simulink model "mcb_microchip_pmsm_parameter_est_SAME70"  (R2023b)
settings: Solver=FixedStepDiscrete  StartTime=0.0  StopTime=15  RelTol=1e-3  EnableMultiTasking=on
InitFcn:
  | mcb_microchip_pmsm_parameter_est_SAME70_data;
values from neighbouring files (symbols this model uses):
  Ts = T_pwm    (= 5e-05)    [mcb_microchip_pmsm_parameter_est_SAME70_data.m]
  Ts_motor = T_pwm/2    (= 2.5e-05)    [mcb_microchip_pmsm_parameter_est_SAME70_data.m]
undefined symbols (not defined in the file or in its folder): A24, AD10, AD7, ADC0, inverter, LQFP144, MaxPer, ms, ns, PA0, PA1, PA10, PA11, PA12, PA13, PA16, PA18, PA9, PB0, PD18, PD19, PD24, PD25, PD26, PI_params, Pin, pmsm, Resol, SAME70Q21B, target, Unsigned
libraries: simulink x18, MCHP_Blockset x13, mcbpmsmparamestlib x5, svdutilitieslib x4, mcbpositiondecoderlib x3, mcbplantlib x1, autolibpmsmexterior x1, mcbcontrolslib x1
(part 4 of 4)

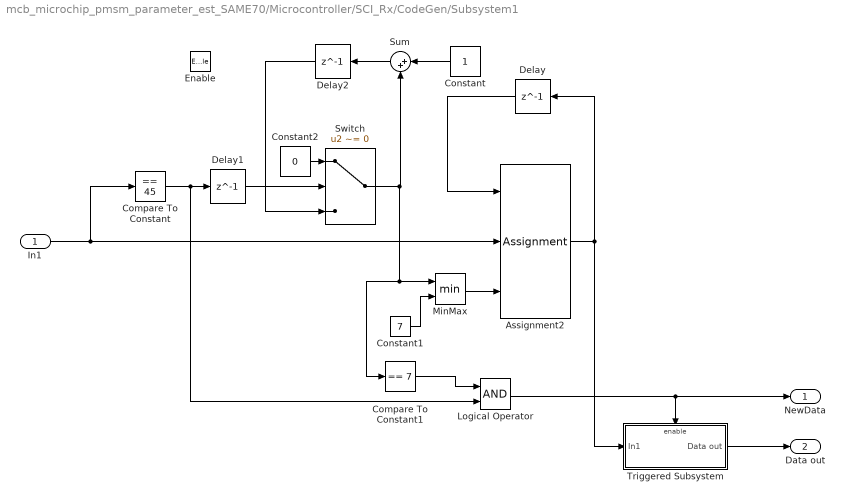
== system mcb_microchip_pmsm_parameter_est_SAME70/Microcontroller/SCI_Rx/CodeGen/Subsystem1 ==
  In1 : Inport
  Enable : EnablePort
  Assignment2 : Assignment  IndexMode=Zero-based  DiagnosticForDimensions=Warning  IndexOptions=Starting index (port)  Indices=1  OutputSizes=1
  Compare To Constant : simulink/Logic and Bit Operations/Compare To Constant  relop===  const=45  OutDataTypeStr=boolean
  Compare To Constant1 : simulink/Logic and Bit Operations/Compare To Constant  relop===  const=7  OutDataTypeStr=boolean
  Constant : Constant  OutDataTypeStr=uint16  SampleTime=-1
  Constant1 : Constant  Value=7  OutDataTypeStr=uint16  SampleTime=-1
  Constant2 : Constant  Value=0  OutDataTypeStr=uint16  SampleTime=-1
  Delay : Delay  DelayLength=1  InitialCondition=[0 0 0 0 0 0 0 0]
  Delay1 : Delay  DelayLength=1  InitialCondition=0
  Delay2 : Delay  DelayLength=1  InitialCondition=0
  Logical Operator : Logic  AllPortsSameDT=off  OutDataTypeStr=boolean
  MinMax : MinMax  Inputs=2
  Sum : Sum  Inputs=|++
  Switch : Switch  Criteria=u2 ~= 0  SaturateOnIntegerOverflow=off  InputSameDT=off
  Triggered Subsystem : Subsystem  TreatAsAtomicUnit=on
  NewData : Outport  OutputWhenDisabled=reset  InitialOutput=0
  Data out : Outport  Port=2
  wires:
  Logical Operator/1 -> Triggered Subsystem/Enable, NewData/1
  Constant2/1 -> Switch/1
  Delay1/1 -> Switch/2
  Switch/1 -> MinMax/1, Compare To Constant1/1, Sum/2
  Sum/1 -> Delay2/1
  MinMax/1 -> Assignment2/3
  Constant1/1 -> MinMax/2
  Constant/1 -> Sum/1
  In1/1 -> Assignment2/2, Compare To Constant/1
  Compare To Constant1/1 -> Logical Operator/1
  Compare To Constant/1 -> Delay1/1, Logical Operator/2
  Delay2/1 -> Switch/3
  Delay/1 -> Assignment2/1
  Assignment2/1 -> Delay/1, Triggered Subsystem/1(In1)
  Triggered Subsystem/1(Data out) -> Data out/1

== system mcb_microchip_pmsm_parameter_est_SAME70/Microcontroller/SCI_Tx/Codegen/Data ==
  Data : Inport
  Action Port : ActionPort  ActionPortLabel=else
  UART Tx : MCHP_Blockset/BUS UART/UART Tx  UART_REF=UART 0  ORDERING=None  AllOrNothing=off  SampleTime=-1  MCHP_MASTERLINK=mcb_microchip_pmsm_parameter_est_SAME70_23b_lib/Microcontroller/Configurations/Microchip Master  NSend_Input=off  UART_String=off  NSend_Output=off
      settings: SourceProductName=MPLAB Device Blocks for Simulink
  wires:
  Data/1 -> UART Tx/1

== system mcb_microchip_pmsm_parameter_est_SAME70/Microcontroller/SCI_Tx/Codegen/End ==
  Data : Inport
  Action Port : ActionPort  ActionPortLabel=elseif(u1 == single(target.SerialFrameSize-1))
  Mux : Mux  Inputs=2
  Start : Constant  Value=hex2dec('45')  OutDataTypeStr=uint8
  UART Tx : MCHP_Blockset/BUS UART/UART Tx  UART_REF=UART 0  ORDERING=None  AllOrNothing=off  SampleTime=-1  MCHP_MASTERLINK=mcb_microchip_pmsm_parameter_est_SAME70_23b_lib/Microcontroller/Configurations/Microchip Master  NSend_Input=off  UART_String=off  NSend_Output=off
      settings: SourceProductName=MPLAB Device Blocks for Simulink
  wires:
  Start/1 -> Mux/2
  Data/1 -> Mux/1
  Mux/1 -> UART Tx/1

== system mcb_microchip_pmsm_parameter_est_SAME70/Microcontroller/SCI_Tx/Codegen/Start ==
  Data : Inport
  Action Port : ActionPort  ActionPortLabel=if(u1 == 0)
  End : Constant  Value=hex2dec('53')  OutDataTypeStr=uint8
  Mux : Mux  Inputs=2
  UART Tx : MCHP_Blockset/BUS UART/UART Tx  UART_REF=UART 0  ORDERING=None  AllOrNothing=off  SampleTime=-1  MCHP_MASTERLINK=mcb_microchip_pmsm_parameter_est_SAME70_23b_lib/Microcontroller/Configurations/Microchip Master  NSend_Input=off  UART_String=off  NSend_Output=off
      settings: SourceProductName=MPLAB Device Blocks for Simulink
  wires:
  End/1 -> Mux/1
  Data/1 -> Mux/2
  Mux/1 -> UART Tx/1

== system mcb_microchip_pmsm_parameter_est_SAME70/Inverter and Motor/Inverter and Motor/Sim/Motor/Inverter ==
  Duty_abc : Inport
  Average-Value Inverter : mcbplantlib/Average-Value Inverter
  Constant2 : Constant  Value=inverter.V_dc  OutDataTypeStr=single  SampleTime=-1
  Data Type Conversion1 : DataTypeConversion  OutDataTypeStr=single  RndMeth=Simplest  SaturateOnIntegerOverflow=off
  Vabc : Outport
  wires:
  Constant2/1 -> Average-Value Inverter/2
  Duty_abc/1 -> Data Type Conversion1/1
  Average-Value Inverter/1 -> Vabc/1
  Data Type Conversion1/1 -> Average-Value Inverter/1

== system mcb_microchip_pmsm_parameter_est_SAME70/Microcontroller/Application/Param Est/MechParam/Select J ==
  Jin : Inport
  codegen : Subsystem  VariantControl=(codegen)
  sim : Subsystem  VariantControl=(sim)
  Jout : Outport

== system mcb_microchip_pmsm_parameter_est_SAME70/Microcontroller/Application Abstraction/Variant Subsystem/Index Absent/Enabled Subsystem ==
  In1 : Inport
  Enable : EnablePort
  Out1 : Outport
  wires:
  In1/1 -> Out1/1

== system mcb_microchip_pmsm_parameter_est_SAME70/Microcontroller/Input HW Drivers/Codegen/Qdec_interface/If Action Subsystem ==
  In1 : Inport
  Action Port : ActionPort  ActionPortLabel=if((u1 > 49151 ) & (u2 < 16384 ))
  Add : Sum
  Constant : Constant  Value=(EnCountPerRev) -mod(65536,(EnCountPerRev))  OutDataTypeStr=uint16
  Out1 : Outport
  wires:
  In1/1 -> Add/1
  Constant/1 -> Add/2
  Add/1 -> Out1/1

== system mcb_microchip_pmsm_parameter_est_SAME70/Microcontroller/Input HW Drivers/Codegen/Qdec_interface/If Action Subsystem1 ==
  In1 : Inport
  Action Port : ActionPort  ActionPortLabel=elseif((u2 > 49151 ) & (u1 < 16384 ))
  Add : Sum
  Constant : Constant  Value=mod(65536,(EnCountPerRev))  OutDataTypeStr=uint16
  Out1 : Outport
  wires:
  Add/1 -> Out1/1
  Constant/1 -> Add/2
  In1/1 -> Add/1

== system mcb_microchip_pmsm_parameter_est_SAME70/Microcontroller/Input HW Drivers/Codegen/Qdec_interface/If Action Subsystem2 ==
  In1 : Inport
  Action Port : ActionPort  ActionPortLabel=else
  Out1 : Outport
  wires:
  In1/1 -> Out1/1

== system mcb_microchip_pmsm_parameter_est_SAME70/Microcontroller/Input HW Drivers/Codegen/Qdec_interface/Offset ==
  QdecCount : Inport
  Enable : EnablePort
  Add1 : Sum  Inputs=-+  OutDataTypeStr=uint16
  Constant2 : Constant  Value=EnCountPerRev  OutDataTypeStr=Inherit: Inherit via back propagation
  Data Store Write : DataStoreWrite  DataStoreName=PosOffset  IndexOptions=Index vector (dialog)  Indices=1  OutputSizes=1
  Math Function1 : Math  Operator=mod  SignedPower=on
  wires:
  QdecCount/1 -> Math Function1/1
  Constant2/1 -> Add1/2, Math Function1/2
  Add1/1 -> Data Store Write/1
  Math Function1/1 -> Add1/1

== system mcb_microchip_pmsm_parameter_est_SAME70/Microcontroller/Input Scaling/Variant Subsystem/Automatic offset calibration/Enabled Subsystem ==
  In1 : Inport
  Enable : EnablePort
  Out1 : Outport
  wires:
  In1/1 -> Out1/1

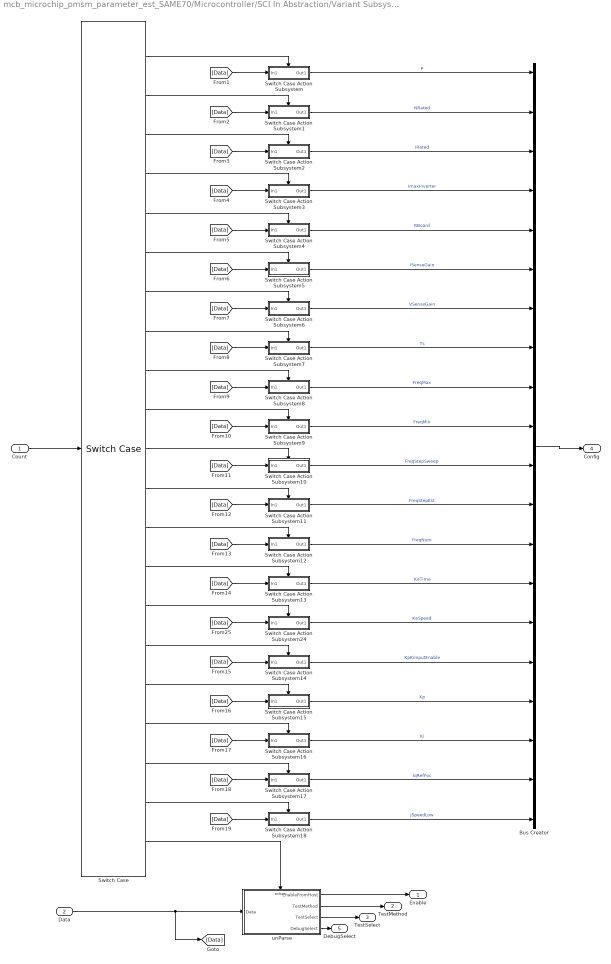
== system mcb_microchip_pmsm_parameter_est_SAME70/Microcontroller/SCI In Abstraction/Variant Subsystem/Codegen/Subsystem1 ==
  Count : Inport
  Data : Inport  Port=2
  Bus Creator : BusCreator  Inputs=20
  Switch Case : SwitchCase  CaseConditions={1 2 3 4 5 6 7 8 9 10 11 12 13 14 15 16 17 18 19 20 21}  ShowDefaultCase=off
  Switch Case Action Subsystem : Subsystem  TreatAsAtomicUnit=on
  Switch Case Action Subsystem1 : Subsystem  TreatAsAtomicUnit=on
  Switch Case Action Subsystem10 : Subsystem  TreatAsAtomicUnit=on
  Switch Case Action Subsystem11 : Subsystem  TreatAsAtomicUnit=on
  Switch Case Action Subsystem12 : Subsystem  TreatAsAtomicUnit=on
  Switch Case Action Subsystem13 : Subsystem  TreatAsAtomicUnit=on
  Switch Case Action Subsystem14 : Subsystem  TreatAsAtomicUnit=on
  Switch Case Action Subsystem15 : Subsystem  TreatAsAtomicUnit=on
  Switch Case Action Subsystem16 : Subsystem  TreatAsAtomicUnit=on
  Switch Case Action Subsystem17 : Subsystem  TreatAsAtomicUnit=on
  Switch Case Action Subsystem18 : Subsystem  TreatAsAtomicUnit=on
  Switch Case Action Subsystem2 : Subsystem  TreatAsAtomicUnit=on
  Switch Case Action Subsystem24 : Subsystem  TreatAsAtomicUnit=on
  Switch Case Action Subsystem3 : Subsystem  TreatAsAtomicUnit=on
  Switch Case Action Subsystem4 : Subsystem  TreatAsAtomicUnit=on
  Switch Case Action Subsystem5 : Subsystem  TreatAsAtomicUnit=on
  Switch Case Action Subsystem6 : Subsystem  TreatAsAtomicUnit=on
  Switch Case Action Subsystem7 : Subsystem  TreatAsAtomicUnit=on
  Switch Case Action Subsystem8 : Subsystem  TreatAsAtomicUnit=on
  Switch Case Action Subsystem9 : Subsystem  TreatAsAtomicUnit=on
  unParse : Subsystem
  Enable : Outport
  TestMethod : Outport  Port=2
  TestSelect : Outport  Port=3
  Config : Outport  Port=4
  DebugSelect : Outport  Port=5
  wires:
  Count/1 -> Switch Case/1
  Data/1 -> [Data], unParse/1(Data)
  unParse/1(EnableFromHost) -> Enable/1
  unParse/2(TestMethod) -> TestMethod/1
  unParse/3(TestSelect) -> TestSelect/1
  Bus Creator/1 -> Config/1
  [Data] -> Switch Case Action Subsystem/1(In1)
  [Data] -> Switch Case Action Subsystem1/1(In1)
  [Data] -> Switch Case Action Subsystem2/1(In1)
  [Data] -> Switch Case Action Subsystem3/1(In1)
  [Data] -> Switch Case Action Subsystem4/1(In1)
  [Data] -> Switch Case Action Subsystem5/1(In1)
  [Data] -> Switch Case Action Subsystem6/1(In1)
  [Data] -> Switch Case Action Subsystem7/1(In1)
  [Data] -> Switch Case Action Subsystem8/1(In1)
  [Data] -> Switch Case Action Subsystem9/1(In1)
  [Data] -> Switch Case Action Subsystem10/1(In1)
  [Data] -> Switch Case Action Subsystem11/1(In1)
  [Data] -> Switch Case Action Subsystem12/1(In1)
  [Data] -> Switch Case Action Subsystem13/1(In1)
  [Data] -> Switch Case Action Subsystem14/1(In1)
  [Data] -> Switch Case Action Subsystem15/1(In1)
  [Data] -> Switch Case Action Subsystem16/1(In1)
  [Data] -> Switch Case Action Subsystem17/1(In1)
  [Data] -> Switch Case Action Subsystem18/1(In1)
  Switch Case Action Subsystem/1(Out1) -> Bus Creator/1  "P"
  Switch Case Action Subsystem1/1(Out1) -> Bus Creator/2  "NRated"
  Switch Case Action Subsystem2/1(Out1) -> Bus Creator/3  "IRated"
  Switch Case Action Subsystem3/1(Out1) -> Bus Creator/4  "ImaxInverter"
  Switch Case Action Subsystem4/1(Out1) -> Bus Creator/5  "RBoard"
  Switch Case Action Subsystem5/1(Out1) -> Bus Creator/6  "ISenseGain"
  Switch Case Action Subsystem6/1(Out1) -> Bus Creator/7  "VSenseGain"
  Switch Case Action Subsystem7/1(Out1) -> Bus Creator/8  "Ts"
  unParse/4(DebugSelect) -> DebugSelect/1
  [Data] -> Switch Case Action Subsystem24/1(In1)
  Switch Case/1 -> Switch Case Action Subsystem/Action
  Switch Case/2 -> Switch Case Action Subsystem1/Action
  Switch Case/3 -> Switch Case Action Subsystem2/Action
  Switch Case/4 -> Switch Case Action Subsystem3/Action
  Switch Case/5 -> Switch Case Action Subsystem4/Action
  Switch Case/6 -> Switch Case Action Subsystem5/Action
  Switch Case/7 -> Switch Case Action Subsystem6/Action
  Switch Case/8 -> Switch Case Action Subsystem7/Action
  Switch Case/21 -> unParse/Action
  Switch Case/9 -> Switch Case Action Subsystem8/Action
  Switch Case/10 -> Switch Case Action Subsystem9/Action
  Switch Case/11 -> Switch Case Action Subsystem10/Action
  Switch Case/12 -> Switch Case Action Subsystem11/Action
  Switch Case/13 -> Switch Case Action Subsystem12/Action
  Switch Case/14 -> Switch Case Action Subsystem13/Action
  Switch Case/15 -> Switch Case Action Subsystem24/Action
  Switch Case/16 -> Switch Case Action Subsystem14/Action
  Switch Case/17 -> Switch Case Action Subsystem15/Action
  Switch Case/18 -> Switch Case Action Subsystem16/Action
  Switch Case/19 -> Switch Case Action Subsystem17/Action
  Switch Case/20 -> Switch Case Action Subsystem18/Action
  Switch Case Action Subsystem8/1(Out1) -> Bus Creator/9  "FreqMax"
  Switch Case Action Subsystem9/1(Out1) -> Bus Creator/10  "FreqMin"
  Switch Case Action Subsystem10/1(Out1) -> Bus Creator/11  "FreqStepSweep"
  Switch Case Action Subsystem11/1(Out1) -> Bus Creator/12  "FreqStepEst"
  Switch Case Action Subsystem12/1(Out1) -> Bus Creator/13  "FreqNum"
  Switch Case Action Subsystem13/1(Out1) -> Bus Creator/14  "KeTime"
  Switch Case Action Subsystem24/1(Out1) -> Bus Creator/15  "KeSpeed"
  Switch Case Action Subsystem14/1(Out1) -> Bus Creator/16  "KpKiInputEnable"
  Switch Case Action Subsystem15/1(Out1) -> Bus Creator/17  "Kp"
  Switch Case Action Subsystem16/1(Out1) -> Bus Creator/18  "Ki"
  Switch Case Action Subsystem17/1(Out1) -> Bus Creator/19  "IqRefFoc"
  Switch Case Action Subsystem18/1(Out1) -> Bus Creator/20  "JSpeedLow"

== system mcb_microchip_pmsm_parameter_est_SAME70/Microcontroller/SCI_Rx/CodeGen/Subsystem1/Triggered Subsystem ==
  In1 : Inport
  Enable : EnablePort
  Data out : Outport
  wires:
  In1/1 -> Data out/1

== system mcb_microchip_pmsm_parameter_est_SAME70/Microcontroller/Application/Param Est/MechParam/Select J/codegen ==
  Jin : Inport
  Jout : Outport
  wires:
  Jin/1 -> Jout/1

== system mcb_microchip_pmsm_parameter_est_SAME70/Microcontroller/Application/Param Est/MechParam/Select J/sim ==
  Jin : Inport
  Constant : Constant  Value=pmsm.J  OutDataTypeStr=Inherit: Inherit via back propagation
  Terminator : Terminator
  Jout : Outport
  wires:
  Jin/1 -> Terminator/1
  Constant/1 -> Jout/1

== system mcb_microchip_pmsm_parameter_est_SAME70/Microcontroller/SCI In Abstraction/Variant Subsystem/Codegen/Subsystem1/Switch Case Action Subsystem ==
  In1 : Inport
  Action Port : ActionPort  ActionPortLabel=case [ 1 ]:
  Out1 : Outport
  wires:
  In1/1 -> Out1/1

== system mcb_microchip_pmsm_parameter_est_SAME70/Microcontroller/SCI In Abstraction/Variant Subsystem/Codegen/Subsystem1/Switch Case Action Subsystem1 ==
  In1 : Inport
  Action Port : ActionPort  ActionPortLabel=case [ 2 ]:
  Out1 : Outport
  wires:
  In1/1 -> Out1/1

== system mcb_microchip_pmsm_parameter_est_SAME70/Microcontroller/SCI In Abstraction/Variant Subsystem/Codegen/Subsystem1/Switch Case Action Subsystem10 ==
  In1 : Inport
  Action Port : ActionPort  ActionPortLabel=case [ 11 ]:
  Out1 : Outport
  wires:
  In1/1 -> Out1/1

== system mcb_microchip_pmsm_parameter_est_SAME70/Microcontroller/SCI In Abstraction/Variant Subsystem/Codegen/Subsystem1/Switch Case Action Subsystem11 ==
  In1 : Inport
  Action Port : ActionPort  ActionPortLabel=case [ 12 ]:
  Out1 : Outport
  wires:
  In1/1 -> Out1/1

== system mcb_microchip_pmsm_parameter_est_SAME70/Microcontroller/SCI In Abstraction/Variant Subsystem/Codegen/Subsystem1/Switch Case Action Subsystem12 ==
  In1 : Inport
  Action Port : ActionPort  ActionPortLabel=case [ 13 ]:
  Out1 : Outport
  wires:
  In1/1 -> Out1/1

== system mcb_microchip_pmsm_parameter_est_SAME70/Microcontroller/SCI In Abstraction/Variant Subsystem/Codegen/Subsystem1/Switch Case Action Subsystem13 ==
  In1 : Inport
  Action Port : ActionPort  ActionPortLabel=case [ 14 ]:
  Out1 : Outport
  wires:
  In1/1 -> Out1/1

== system mcb_microchip_pmsm_parameter_est_SAME70/Microcontroller/SCI In Abstraction/Variant Subsystem/Codegen/Subsystem1/Switch Case Action Subsystem14 ==
  In1 : Inport
  Action Port : ActionPort  ActionPortLabel=case [ 16 ]:
  Out1 : Outport
  wires:
  In1/1 -> Out1/1

== system mcb_microchip_pmsm_parameter_est_SAME70/Microcontroller/SCI In Abstraction/Variant Subsystem/Codegen/Subsystem1/Switch Case Action Subsystem15 ==
  In1 : Inport
  Action Port : ActionPort  ActionPortLabel=case [ 17 ]:
  Out1 : Outport
  wires:
  In1/1 -> Out1/1

== system mcb_microchip_pmsm_parameter_est_SAME70/Microcontroller/SCI In Abstraction/Variant Subsystem/Codegen/Subsystem1/Switch Case Action Subsystem16 ==
  In1 : Inport
  Action Port : ActionPort  ActionPortLabel=case [ 18 ]:
  Out1 : Outport
  wires:
  In1/1 -> Out1/1

== system mcb_microchip_pmsm_parameter_est_SAME70/Microcontroller/SCI In Abstraction/Variant Subsystem/Codegen/Subsystem1/Switch Case Action Subsystem17 ==
  In1 : Inport
  Action Port : ActionPort  ActionPortLabel=case [ 19 ]:
  Out1 : Outport
  wires:
  In1/1 -> Out1/1

== system mcb_microchip_pmsm_parameter_est_SAME70/Microcontroller/SCI In Abstraction/Variant Subsystem/Codegen/Subsystem1/Switch Case Action Subsystem18 ==
  In1 : Inport
  Action Port : ActionPort  ActionPortLabel=case [ 20 ]:
  Out1 : Outport
  wires:
  In1/1 -> Out1/1

== system mcb_microchip_pmsm_parameter_est_SAME70/Microcontroller/SCI In Abstraction/Variant Subsystem/Codegen/Subsystem1/Switch Case Action Subsystem2 ==
  In1 : Inport
  Action Port : ActionPort  ActionPortLabel=case [ 3 ]:
  Out1 : Outport
  wires:
  In1/1 -> Out1/1

== system mcb_microchip_pmsm_parameter_est_SAME70/Microcontroller/SCI In Abstraction/Variant Subsystem/Codegen/Subsystem1/Switch Case Action Subsystem24 ==
  In1 : Inport
  Action Port : ActionPort  ActionPortLabel=case [ 15 ]:
  Out1 : Outport
  wires:
  In1/1 -> Out1/1

== system mcb_microchip_pmsm_parameter_est_SAME70/Microcontroller/SCI In Abstraction/Variant Subsystem/Codegen/Subsystem1/Switch Case Action Subsystem3 ==
  In1 : Inport
  Action Port : ActionPort  ActionPortLabel=case [ 4 ]:
  Out1 : Outport
  wires:
  In1/1 -> Out1/1

== system mcb_microchip_pmsm_parameter_est_SAME70/Microcontroller/SCI In Abstraction/Variant Subsystem/Codegen/Subsystem1/Switch Case Action Subsystem4 ==
  In1 : Inport
  Action Port : ActionPort  ActionPortLabel=case [ 5 ]:
  Out1 : Outport
  wires:
  In1/1 -> Out1/1

== system mcb_microchip_pmsm_parameter_est_SAME70/Microcontroller/SCI In Abstraction/Variant Subsystem/Codegen/Subsystem1/Switch Case Action Subsystem5 ==
  In1 : Inport
  Action Port : ActionPort  ActionPortLabel=case [ 6 ]:
  Out1 : Outport
  wires:
  In1/1 -> Out1/1

== system mcb_microchip_pmsm_parameter_est_SAME70/Microcontroller/SCI In Abstraction/Variant Subsystem/Codegen/Subsystem1/Switch Case Action Subsystem6 ==
  In1 : Inport
  Action Port : ActionPort  ActionPortLabel=case [ 7 ]:
  Out1 : Outport
  wires:
  In1/1 -> Out1/1

== system mcb_microchip_pmsm_parameter_est_SAME70/Microcontroller/SCI In Abstraction/Variant Subsystem/Codegen/Subsystem1/Switch Case Action Subsystem7 ==
  In1 : Inport
  Action Port : ActionPort  ActionPortLabel=case [ 8 ]:
  Out1 : Outport
  wires:
  In1/1 -> Out1/1

== system mcb_microchip_pmsm_parameter_est_SAME70/Microcontroller/SCI In Abstraction/Variant Subsystem/Codegen/Subsystem1/Switch Case Action Subsystem8 ==
  In1 : Inport
  Action Port : ActionPort  ActionPortLabel=case [ 9 ]:
  Out1 : Outport
  wires:
  In1/1 -> Out1/1

== system mcb_microchip_pmsm_parameter_est_SAME70/Microcontroller/SCI In Abstraction/Variant Subsystem/Codegen/Subsystem1/Switch Case Action Subsystem9 ==
  In1 : Inport
  Action Port : ActionPort  ActionPortLabel=case [ 10 ]:
  Out1 : Outport
  wires:
  In1/1 -> Out1/1

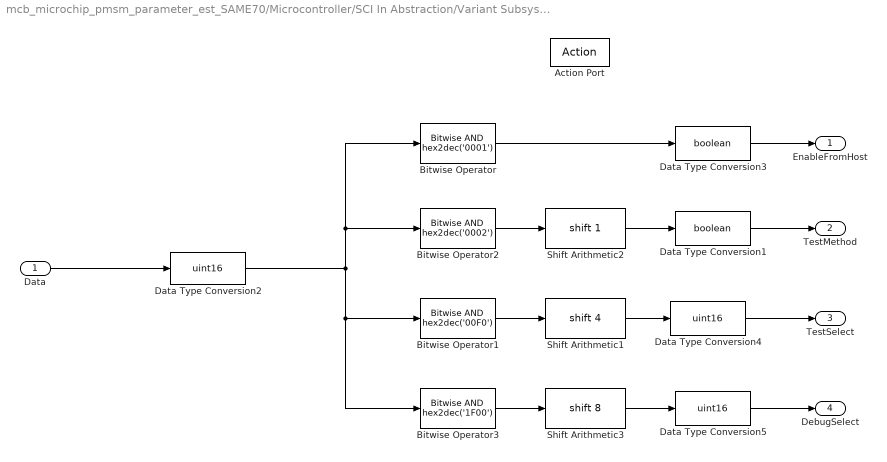
== system mcb_microchip_pmsm_parameter_est_SAME70/Microcontroller/SCI In Abstraction/Variant Subsystem/Codegen/Subsystem1/unParse ==
  Data : Inport
  Action Port : ActionPort  ActionPortLabel=case [ 21 ]:
  Bitwise Operator : simulink/Logic and Bit Operations/Bitwise Operator  logicop=AND  UseBitMask=on  BitMask=hex2dec('0001')  BitMaskRealWorld=Stored Integer
  Bitwise Operator1 : simulink/Logic and Bit Operations/Bitwise Operator  logicop=AND  UseBitMask=on  BitMask=hex2dec('00F0')  BitMaskRealWorld=Stored Integer
  Bitwise Operator2 : simulink/Logic and Bit Operations/Bitwise Operator  logicop=AND  UseBitMask=on  BitMask=hex2dec('0002')  BitMaskRealWorld=Stored Integer
  Bitwise Operator3 : simulink/Logic and Bit Operations/Bitwise Operator  logicop=AND  UseBitMask=on  BitMask=hex2dec('1F00')  BitMaskRealWorld=Stored Integer
  Data Type Conversion1 : DataTypeConversion  OutDataTypeStr=boolean  RndMeth=Simplest  SaturateOnIntegerOverflow=off
  Data Type Conversion2 : DataTypeConversion  OutDataTypeStr=uint16  RndMeth=Simplest  SaturateOnIntegerOverflow=off
  Data Type Conversion3 : DataTypeConversion  OutDataTypeStr=boolean  RndMeth=Simplest  SaturateOnIntegerOverflow=off
  Data Type Conversion4 : DataTypeConversion  OutDataTypeStr=uint16  RndMeth=Simplest  SaturateOnIntegerOverflow=off
  Data Type Conversion5 : DataTypeConversion  OutDataTypeStr=uint16  RndMeth=Simplest  SaturateOnIntegerOverflow=off
  Shift Arithmetic1 : ArithShift  BitShiftNumber=4
  Shift Arithmetic2 : ArithShift  BitShiftNumber=1
  Shift Arithmetic3 : ArithShift  BitShiftNumber=8
  EnableFromHost : Outport
  TestMethod : Outport  Port=2
  TestSelect : Outport  Port=3
  DebugSelect : Outport  Port=4
  wires:
  Data Type Conversion1/1 -> TestMethod/1
  Shift Arithmetic2/1 -> Data Type Conversion1/1
  Bitwise Operator2/1 -> Shift Arithmetic2/1
  Data Type Conversion3/1 -> EnableFromHost/1
  Shift Arithmetic1/1 -> Data Type Conversion4/1
  Data Type Conversion4/1 -> TestSelect/1
  Bitwise Operator/1 -> Data Type Conversion3/1
  Data/1 -> Data Type Conversion2/1
  Bitwise Operator1/1 -> Shift Arithmetic1/1
  Data Type Conversion2/1 -> Bitwise Operator2/1, Bitwise Operator/1, Bitwise Operator3/1, Bitwise Operator1/1
  Bitwise Operator3/1 -> Shift Arithmetic3/1
  Data Type Conversion5/1 -> DebugSelect/1
  Shift Arithmetic3/1 -> Data Type Conversion5/1

== stateflow chart mcb_microchip_pmsm_parameter_est_SAME70/Microcontroller/Application/Param Est/Test Control/Chart ==
  state Init
    during: TestNum = uint16(0);
  state RsTestState
    during: TestNum = uint16(1);
  state LdTestState
    during: TestNum = uint16(2);
  state LqTestState1
    during: TestNum = uint16(3);
  state MechTestState
    during: TestNum = uint16(4);
  RsTestState -> Init [order 2] : [EnableIn == 0]
  (default) -> Init
  Init -> RsTestState : [EnableIn == 1 && EnPrev == 0]
  RsTestState -> LdTestState [order 1] : after(1/Ts,tick)[RsStatus == 2]
  MechTestState -> Init : after(1/Ts,tick)[MechStatus == 2]
  LqTestState1 -> Init [order 2] : [EnableIn == 0]
  LdTestState -> Init [order 2] : [EnableIn == 0]
  LdTestState -> LqTestState1 [order 1] : after(1/Ts,tick)[LdStatus == 2]
  LqTestState1 -> MechTestState [order 1] : after(1/Ts,tick)[LqStatus == 2]
  data: TestNum output; EnableIn input; EnPrev input; RsStatus input; LdStatus input; LqStatus input; MechStatus input; Ts input
